simulink model "beisp_5"  (Simulink 3.00)
settings: Solver=FixedStepDiscrete  SolverMode=SingleTasking  StartTime=0.0  StopTime=10.0  FixedStep=Ts  RelTol=1e-3  AbsTol=1e-6
values from neighbouring files (symbols this model uses):
  Ts = 0.5    [mehrw_4.m]    (also in mehrw_5.m; pbeisp_5.m = 0.1)
undefined symbols (not defined in the file or in its folder): ad, bd
libraries: simulink3 x1
settings Model: LoadExternalInput=on  ExternalInput=A1

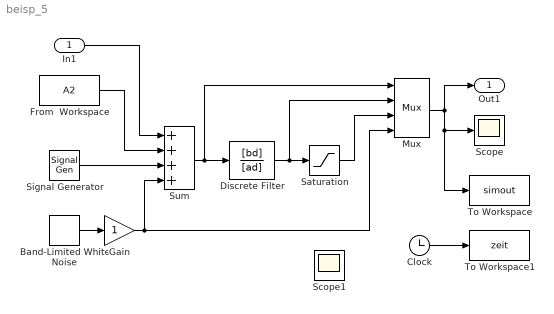
== system beisp_5 ==
  In1 : Inport  Port=1  PortWidth=-1  SampleTime=-1  DataType=auto
      settings: SignalType=auto
  Band-Limited White Noise : simulink3/Sources/Band-Limited White Noise  Cov=[Ts]  Ts=Ts  seed=[23341]
  Clock : Clock
      settings: DisplayTime=off  Decimation=10
  Discrete Filter : DiscreteFilter  Numerator=[bd]  Denominator=[ad]  SampleTime=Ts
  From  Workspace : FromWorkspace  VariableName=A2  SampleTime=0  HoldFinalValue=off
  Gain : Gain  Gain=1  SaturateOnIntegerOverflow=on
  Mux : Mux  Inputs=4
      settings: DisplayOption=none
  Saturation : Saturate  UpperLimit=4.5  LowerLimit=-4.5
  Scope : Scope
      settings: TickLabels=on  TimeRange=auto  YMin=-5  YMax=5  SaveToWorkspace=off  SaveName=ScopeData  DataFormat=Matrix
  Scope1 : Scope
      settings: Floating=on  TickLabels=on  TimeRange=auto  YMin=-5  YMax=5  SaveToWorkspace=off  SaveName=ScopeData  DataFormat=Matrix
  Signal Generator : SignalGenerator  WaveForm=square  Amplitude=5  Frequency=0.15  Units=Hertz
  Sum : Sum  Inputs=++++  SaturateOnIntegerOverflow=on
  To Workspace : ToWorkspace  VariableName=simout  SampleTime=-1  SaveFormat=Matrix
      settings: Buffer=1000
  To Workspace1 : ToWorkspace  VariableName=zeit  SampleTime=-1  SaveFormat=Matrix
      settings: Buffer=1000
  Out1 : Outport  Port=1
  wires:
  Signal Generator/1 -> Sum/3
  From  Workspace/1 -> Sum/2
  Band-Limited White Noise/1 -> Gain/1
  Saturation/1 -> Mux/3
  Sum/1 -> Discrete Filter/1, Mux/1
  Discrete Filter/1 -> Saturation/1, Mux/2
  In1/1 -> Sum/1
  Gain/1 -> Sum/4, Mux/4
  Mux/1 -> Out1/1, To Workspace/1, Scope/1
  Clock/1 -> To Workspace1/1
